simulink model "UAV_Simulation"  (R2021a)
settings: Solver=VariableStepAuto  StartTime=0.0  StopTime=100  RelTol=1e-3
libraries: pid_lib x4
settings Model: Creator=ewert  LastModifiedBy=varsh
settings SolverCC: AlgebraicLoopSolver=TrustRegion
settings DataIOCC: ReturnWorkspaceOutputs=off
settings DebuggingCC: SFMachineParentedDataDiag=warning  ArithmeticOperatorsInVariantConditions=warning
settings SFSimCC: SimUseLocalCustomCode=off  CustomCodeUndefinedFunction=UseInterfaceOnly
settings RTWCC: RTWUseLocalCustomCode=off
settings CodeAppCC: StateflowObjectComments=on

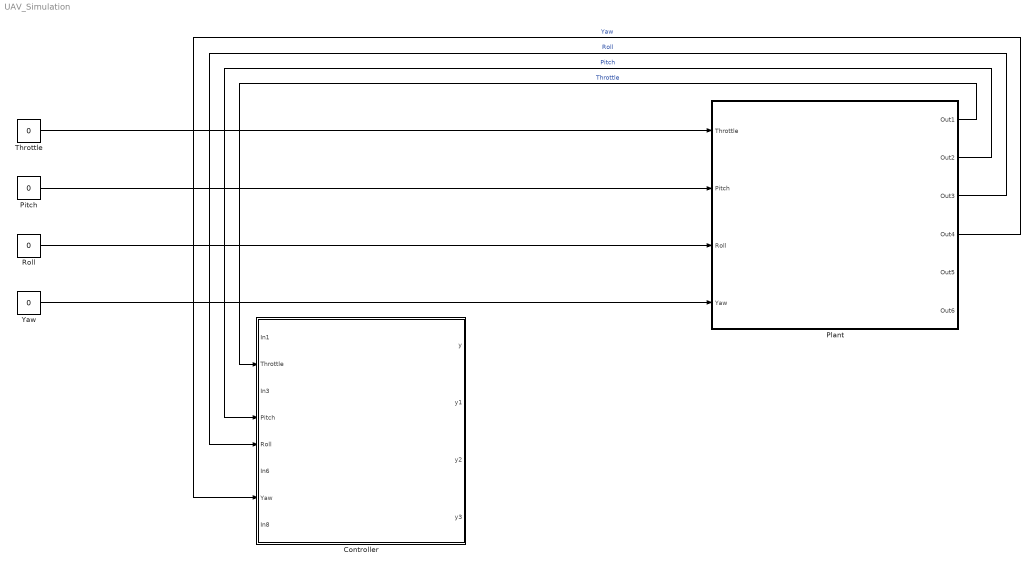
== system UAV_Simulation ==
  Controller : Subsystem
  Pitch : Constant  Value=0
  Plant : Subsystem
  Roll : Constant  Value=0
  Throttle : Constant  Value=0
  Yaw : Constant  Value=0
  wires:
  Plant/1(Out1) -> Controller/2(Throttle)  "Throttle"
  Plant/2(Out2) -> Controller/4(Pitch)  "Pitch"
  Plant/3(Out3) -> Controller/5(Roll)  "Roll"
  Plant/4(Out4) -> Controller/7(Yaw)  "Yaw"
  Roll/1 -> Plant/3(Roll)
  Yaw/1 -> Plant/4(Yaw)
  Throttle/1 -> Plant/1(Throttle)
  Pitch/1 -> Plant/2(Pitch)

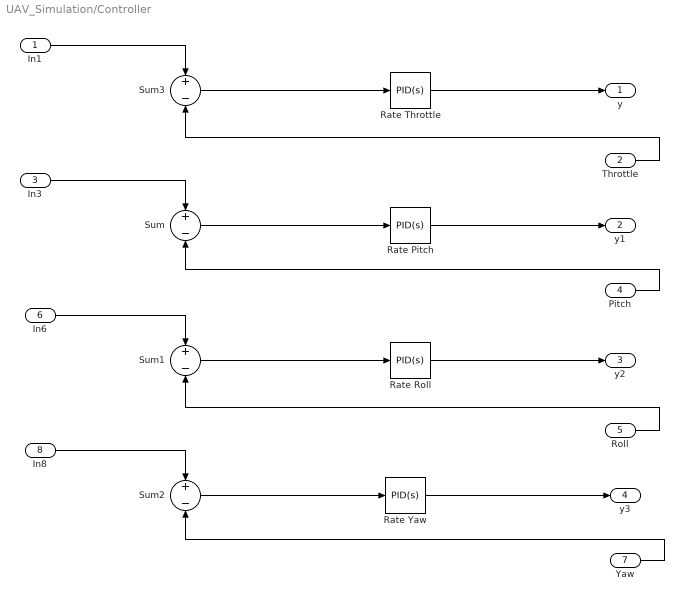
== system UAV_Simulation/Controller ==
  In1 : Inport
  Throttle : Inport  Port=2
  In3 : Inport  Port=3
  Pitch : Inport  Port=4
  Roll : Inport  Port=5
  In6 : Inport  Port=6
  Yaw : Inport  Port=7
  In8 : Inport  Port=8
  Rate Pitch : pid_lib/PID Controller  Controller=PID  Form=Parallel  TimeDomain=Continuous-time  UseExternalTs=off  SampleTime=-1  IntegratorMethod=Forward Euler  FilterMethod=Forward Euler  ControllerParametersSource=internal  P=5  I=1  D=0  UseFilter=on  N=100  TunerSelectOption=Transfer Function Based (PID Tuner App)  InitialConditionSource=internal  InitialConditionForIntegrator=0  InitialConditionForFilter=0  DifferentiatorICPrevScaledInput=0  ExternalReset=none  TrackingMode=off  Kt=1  LimitOutput=on  SatLimitsSource=internal  UpperSaturationLimit=100  LowerSaturationLimit=0  LinearizeAsGain=on  AntiWindupMode=clamping  Kb=1  POutMin=[]  POutMax=[]  IOutMin=[]  IOutMax=[]  DOutMin=[]  DOutMax=[]  NOutMin=[]  NOutMax=[]  SumOutMin=[]  SumOutMax=[]  SaturationOutMin=[]  SaturationOutMax=[]  PParamMin=[]  PParamMax=[]  IParamMin=[]  IParamMax=[]  DParamMin=[]  DParamMax=[]  NParamMin=[]  NParamMax=[]  KbParamMin=[]  KbParamMax=[]  KtParamMin=[]  KtParamMax=[]  KbOutMin=[]  KbOutMax=[]  KtOutMin=[]  KtOutMax=[]  IntegratorOutMin=[]  IntegratorOutMax=[]  FilterOutMin=[]  FilterOutMax=[]  SumI1OutMin=[]  SumI1OutMax=[]  SumI2OutMin=[]  SumI2OutMax=[]  SumI3OutMin=[]  SumI3OutMax=[]  SumI4OutMin=[]  SumI4OutMax=[]  SumDOutMin=[]  SumDOutMax=[]  DifferentiatorOutMin=[]  DifferentiatorOutMax=[]  FilterDiffOutCoefMin=[]  FilterDiffOutCoefMax=[]  ReciprocalOutMin=[]  ReciprocalOutMax=[]  SumDenOutMin=[]  SumDenOutMax=[]  SumNumOutMin=[]  SumNumOutMax=[]  DivideOutMin=[]  DivideOutMax=[]  UdiffTsProdOutMin=[]  UdiffTsProdOutMax=[]  NTsProdOutMin=[]  NTsProdOutMax=[]  UintegralTsProdOutMin=[]  UintegralTsProdOutMax=[]  UngainTsProdOutMin=[]  UngainTsProdOutMax=[]  IntegratorContinuousStateAttributes=''  IntegratorStateMustResolveToSignalObject=off  IntegratorRTWStateStorageClass=Auto  FilterContinuousStateAttributes=''  FilterStateMustResolveToSignalObject=off  FilterRTWStateStorageClass=Auto  ParallelPVariant=InternalParameters  IdealPVariant=Disabled  IVariant=InternalParameters  DVariant=InternalParameters  IntegratorVariant=Continuous  SatVariant=Enabled  AWVariant=ContClampingParallel  PCopyVariant=Disabled  TRVariant=Disabled  FdbkBlocksVariant=Forward  IdealPFdbkVariant=Disabled  SatFdbkVariant=Disabled  DerivativeFilterVariant=ContFilter  NVariant=InternalParameters  NCopyVariant=Disabled  FilterICVariant=InternalICsFilter  IntegratorICVariant=InternalICs  ExternalResetVariant=Disabled  TRSumVariant=Passthrough  SumFdbkVariant=Disabled  SumVariant=Sum_PID  TsampFilterVariant=InternalTs  TsampNgainVariant=Passthrough  TsampIntegralVariant=Passthrough  ExternalSaturationOutDataTypeStr=Inherit: Same as second input
  Rate Roll : pid_lib/PID Controller  Controller=PID  Form=Parallel  TimeDomain=Continuous-time  UseExternalTs=off  SampleTime=-1  IntegratorMethod=Forward Euler  FilterMethod=Forward Euler  ControllerParametersSource=internal  P=10  I=5  D=0  UseFilter=on  N=100  TunerSelectOption=Transfer Function Based (PID Tuner App)  InitialConditionSource=internal  InitialConditionForIntegrator=0  InitialConditionForFilter=0  DifferentiatorICPrevScaledInput=0  ExternalReset=none  TrackingMode=off  Kt=1  LimitOutput=on  SatLimitsSource=internal  UpperSaturationLimit=100  LowerSaturationLimit=0  LinearizeAsGain=on  AntiWindupMode=clamping  Kb=1  POutMin=[]  POutMax=[]  IOutMin=[]  IOutMax=[]  DOutMin=[]  DOutMax=[]  NOutMin=[]  NOutMax=[]  SumOutMin=[]  SumOutMax=[]  SaturationOutMin=[]  SaturationOutMax=[]  PParamMin=[]  PParamMax=[]  IParamMin=[]  IParamMax=[]  DParamMin=[]  DParamMax=[]  NParamMin=[]  NParamMax=[]  KbParamMin=[]  KbParamMax=[]  KtParamMin=[]  KtParamMax=[]  KbOutMin=[]  KbOutMax=[]  KtOutMin=[]  KtOutMax=[]  IntegratorOutMin=[]  IntegratorOutMax=[]  FilterOutMin=[]  FilterOutMax=[]  SumI1OutMin=[]  SumI1OutMax=[]  SumI2OutMin=[]  SumI2OutMax=[]  SumI3OutMin=[]  SumI3OutMax=[]  SumI4OutMin=[]  SumI4OutMax=[]  SumDOutMin=[]  SumDOutMax=[]  DifferentiatorOutMin=[]  DifferentiatorOutMax=[]  FilterDiffOutCoefMin=[]  FilterDiffOutCoefMax=[]  ReciprocalOutMin=[]  ReciprocalOutMax=[]  SumDenOutMin=[]  SumDenOutMax=[]  SumNumOutMin=[]  SumNumOutMax=[]  DivideOutMin=[]  DivideOutMax=[]  UdiffTsProdOutMin=[]  UdiffTsProdOutMax=[]  NTsProdOutMin=[]  NTsProdOutMax=[]  UintegralTsProdOutMin=[]  UintegralTsProdOutMax=[]  UngainTsProdOutMin=[]  UngainTsProdOutMax=[]  IntegratorContinuousStateAttributes=''  IntegratorStateMustResolveToSignalObject=off  IntegratorRTWStateStorageClass=Auto  FilterContinuousStateAttributes=''  FilterStateMustResolveToSignalObject=off  FilterRTWStateStorageClass=Auto  ParallelPVariant=InternalParameters  IdealPVariant=Disabled  IVariant=InternalParameters  DVariant=InternalParameters  IntegratorVariant=Continuous  SatVariant=Enabled  AWVariant=ContClampingParallel  PCopyVariant=Disabled  TRVariant=Disabled  FdbkBlocksVariant=Forward  IdealPFdbkVariant=Disabled  SatFdbkVariant=Disabled  DerivativeFilterVariant=ContFilter  NVariant=InternalParameters  NCopyVariant=Disabled  FilterICVariant=InternalICsFilter  IntegratorICVariant=InternalICs  ExternalResetVariant=Disabled  TRSumVariant=Passthrough  SumFdbkVariant=Disabled  SumVariant=Sum_PID  TsampFilterVariant=InternalTs  TsampNgainVariant=Passthrough  TsampIntegralVariant=Passthrough  ExternalSaturationOutDataTypeStr=Inherit: Same as second input
  Rate Throttle : pid_lib/PID Controller  Controller=PID  Form=Parallel  TimeDomain=Continuous-time  UseExternalTs=off  SampleTime=-1  IntegratorMethod=Forward Euler  FilterMethod=Forward Euler  ControllerParametersSource=internal  P=23.2003030381999  I=0.891787568643448  D=34.3816922508907  UseFilter=on  N=1142.8279760416  TunerSelectOption=Transfer Function Based (PID Tuner App)  InitialConditionSource=internal  InitialConditionForIntegrator=0  InitialConditionForFilter=0  DifferentiatorICPrevScaledInput=0  ExternalReset=none  TrackingMode=off  Kt=1  LimitOutput=on  SatLimitsSource=internal  UpperSaturationLimit=100  LowerSaturationLimit=0  LinearizeAsGain=on  AntiWindupMode=clamping  Kb=1  POutMin=[]  POutMax=[]  IOutMin=[]  IOutMax=[]  DOutMin=[]  DOutMax=[]  NOutMin=[]  NOutMax=[]  SumOutMin=[]  SumOutMax=[]  SaturationOutMin=[]  SaturationOutMax=[]  PParamMin=[]  PParamMax=[]  IParamMin=[]  IParamMax=[]  DParamMin=[]  DParamMax=[]  NParamMin=[]  NParamMax=[]  KbParamMin=[]  KbParamMax=[]  KtParamMin=[]  KtParamMax=[]  KbOutMin=[]  KbOutMax=[]  KtOutMin=[]  KtOutMax=[]  IntegratorOutMin=[]  IntegratorOutMax=[]  FilterOutMin=[]  FilterOutMax=[]  SumI1OutMin=[]  SumI1OutMax=[]  SumI2OutMin=[]  SumI2OutMax=[]  SumI3OutMin=[]  SumI3OutMax=[]  SumI4OutMin=[]  SumI4OutMax=[]  SumDOutMin=[]  SumDOutMax=[]  DifferentiatorOutMin=[]  DifferentiatorOutMax=[]  FilterDiffOutCoefMin=[]  FilterDiffOutCoefMax=[]  ReciprocalOutMin=[]  ReciprocalOutMax=[]  SumDenOutMin=[]  SumDenOutMax=[]  SumNumOutMin=[]  SumNumOutMax=[]  DivideOutMin=[]  DivideOutMax=[]  UdiffTsProdOutMin=[]  UdiffTsProdOutMax=[]  NTsProdOutMin=[]  NTsProdOutMax=[]  UintegralTsProdOutMin=[]  UintegralTsProdOutMax=[]  UngainTsProdOutMin=[]  UngainTsProdOutMax=[]  IntegratorContinuousStateAttributes=''  IntegratorStateMustResolveToSignalObject=off  IntegratorRTWStateStorageClass=Auto  FilterContinuousStateAttributes=''  FilterStateMustResolveToSignalObject=off  FilterRTWStateStorageClass=Auto  ParallelPVariant=InternalParameters  IdealPVariant=Disabled  IVariant=InternalParameters  DVariant=InternalParameters  IntegratorVariant=Continuous  SatVariant=Enabled  AWVariant=ContClampingParallel  PCopyVariant=Disabled  TRVariant=Disabled  FdbkBlocksVariant=Forward  IdealPFdbkVariant=Disabled  SatFdbkVariant=Disabled  DerivativeFilterVariant=ContFilter  NVariant=InternalParameters  NCopyVariant=Disabled  FilterICVariant=InternalICsFilter  IntegratorICVariant=InternalICs  ExternalResetVariant=Disabled  TRSumVariant=Passthrough  SumFdbkVariant=Disabled  SumVariant=Sum_PID  TsampFilterVariant=InternalTs  TsampNgainVariant=Passthrough  TsampIntegralVariant=Passthrough  ExternalSaturationOutDataTypeStr=Inherit: Same as second input
  Rate Yaw : pid_lib/PID Controller  Controller=PID  Form=Parallel  TimeDomain=Continuous-time  UseExternalTs=off  SampleTime=-1  IntegratorMethod=Forward Euler  FilterMethod=Forward Euler  ControllerParametersSource=internal  P=10  I=5  D=0  UseFilter=on  N=100  TunerSelectOption=Transfer Function Based (PID Tuner App)  InitialConditionSource=internal  InitialConditionForIntegrator=0  InitialConditionForFilter=0  DifferentiatorICPrevScaledInput=0  ExternalReset=none  TrackingMode=off  Kt=1  LimitOutput=on  SatLimitsSource=internal  UpperSaturationLimit=100  LowerSaturationLimit=0  LinearizeAsGain=on  AntiWindupMode=clamping  Kb=1  POutMin=[]  POutMax=[]  IOutMin=[]  IOutMax=[]  DOutMin=[]  DOutMax=[]  NOutMin=[]  NOutMax=[]  SumOutMin=[]  SumOutMax=[]  SaturationOutMin=[]  SaturationOutMax=[]  PParamMin=[]  PParamMax=[]  IParamMin=[]  IParamMax=[]  DParamMin=[]  DParamMax=[]  NParamMin=[]  NParamMax=[]  KbParamMin=[]  KbParamMax=[]  KtParamMin=[]  KtParamMax=[]  KbOutMin=[]  KbOutMax=[]  KtOutMin=[]  KtOutMax=[]  IntegratorOutMin=[]  IntegratorOutMax=[]  FilterOutMin=[]  FilterOutMax=[]  SumI1OutMin=[]  SumI1OutMax=[]  SumI2OutMin=[]  SumI2OutMax=[]  SumI3OutMin=[]  SumI3OutMax=[]  SumI4OutMin=[]  SumI4OutMax=[]  SumDOutMin=[]  SumDOutMax=[]  DifferentiatorOutMin=[]  DifferentiatorOutMax=[]  FilterDiffOutCoefMin=[]  FilterDiffOutCoefMax=[]  ReciprocalOutMin=[]  ReciprocalOutMax=[]  SumDenOutMin=[]  SumDenOutMax=[]  SumNumOutMin=[]  SumNumOutMax=[]  DivideOutMin=[]  DivideOutMax=[]  UdiffTsProdOutMin=[]  UdiffTsProdOutMax=[]  NTsProdOutMin=[]  NTsProdOutMax=[]  UintegralTsProdOutMin=[]  UintegralTsProdOutMax=[]  UngainTsProdOutMin=[]  UngainTsProdOutMax=[]  IntegratorContinuousStateAttributes=''  IntegratorStateMustResolveToSignalObject=off  IntegratorRTWStateStorageClass=Auto  FilterContinuousStateAttributes=''  FilterStateMustResolveToSignalObject=off  FilterRTWStateStorageClass=Auto  ParallelPVariant=InternalParameters  IdealPVariant=Disabled  IVariant=InternalParameters  DVariant=InternalParameters  IntegratorVariant=Continuous  SatVariant=Enabled  AWVariant=ContClampingParallel  PCopyVariant=Disabled  TRVariant=Disabled  FdbkBlocksVariant=Forward  IdealPFdbkVariant=Disabled  SatFdbkVariant=Disabled  DerivativeFilterVariant=ContFilter  NVariant=InternalParameters  NCopyVariant=Disabled  FilterICVariant=InternalICsFilter  IntegratorICVariant=InternalICs  ExternalResetVariant=Disabled  TRSumVariant=Passthrough  SumFdbkVariant=Disabled  SumVariant=Sum_PID  TsampFilterVariant=InternalTs  TsampNgainVariant=Passthrough  TsampIntegralVariant=Passthrough  ExternalSaturationOutDataTypeStr=Inherit: Same as second input
  Sum{,1..3} (4 alike) : Sum  Inputs=+-
  y : Outport
  y1 : Outport  Port=2
  y2 : Outport  Port=3
  y3 : Outport  Port=4
  wires:
  Rate Pitch/1 -> y1/1
  Sum/1 -> Rate Pitch/1
  Roll/1 -> Sum1/2
  In6/1 -> Sum1/1
  Sum1/1 -> Rate Roll/1
  Sum2/1 -> Rate Yaw/1
  In8/1 -> Sum2/1
  In3/1 -> Sum/1
  Sum3/1 -> Rate Throttle/1
  Rate Yaw/1 -> y3/1
  Rate Throttle/1 -> y/1
  Rate Roll/1 -> y2/1
  Yaw/1 -> Sum2/2
  Pitch/1 -> Sum/2
  In1/1 -> Sum3/1
  Throttle/1 -> Sum3/2

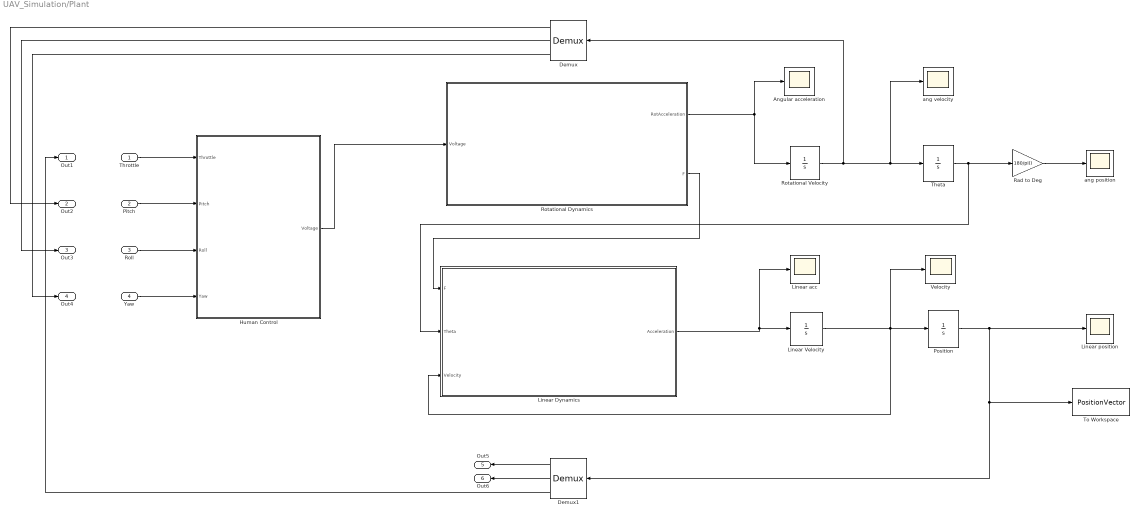
== system UAV_Simulation/Plant ==
  Throttle : Inport
  Pitch : Inport  Port=2
  Roll : Inport  Port=3
  Yaw : Inport  Port=4
  Angular acceleration : Scope
  Demux : Demux  Outputs=3
  Demux1 : Demux  Outputs=3
  Human Control : MATLAB Function  TreatAsAtomicUnit=on
  Linear Dynamics : Subsystem
  Linear Velocity : Integrator
  Linear acc : Scope
  Linear position : Scope
  Position : Integrator
  Rad to Deg : Gain  Gain=180/pi()
  Rotational Dynamics : Subsystem
  Rotational Velocity : Integrator
  Theta : Integrator
  To Workspace : ToWorkspace  VariableName=PositionVector  SampleTime=-1
      settings: Save2DSignal=2-D array (concatenate along first dimension)
  "Velocity " : Scope
  ang position : Scope
  ang velocity : Scope
  Out1 : Outport
  Out2 : Outport  Port=2
  Out3 : Outport  Port=3
  Out4 : Outport  Port=4
  Out5 : Outport  Port=5
  Out6 : Outport  Port=6
  wires:
  Linear Velocity/1 -> Linear Dynamics/3(Velocity), Position/1, "Velocity "/1
  Throttle/1 -> Human Control/1(Throttle)
  Demux1/1 -> Out5/1
  Demux/2 -> Out3/1
  Rotational Velocity/1 -> Theta/1, ang velocity/1, Demux/1
  Position/1 -> Demux1/1, To Workspace/1, Linear position/1
  Theta/1 -> Linear Dynamics/2(Theta), Rad to Deg/1
  Rad to Deg/1 -> ang position/1
  Pitch/1 -> Human Control/2(Pitch)
  Demux/1 -> Out2/1
  Demux1/3 -> Out1/1
  Roll/1 -> Human Control/3(Roll)
  Yaw/1 -> Human Control/4(Yaw)
  Demux/3 -> Out4/1
  Demux1/2 -> Out6/1
  Rotational Dynamics/1(RotAcceleration) -> Rotational Velocity/1, Angular acceleration/1
  Human Control/1(Voltage) -> Rotational Dynamics/1(Voltage)
  Linear Dynamics/1(Acceleration) -> Linear acc/1, Linear Velocity/1
  Rotational Dynamics/2(F) -> Linear Dynamics/1(F)

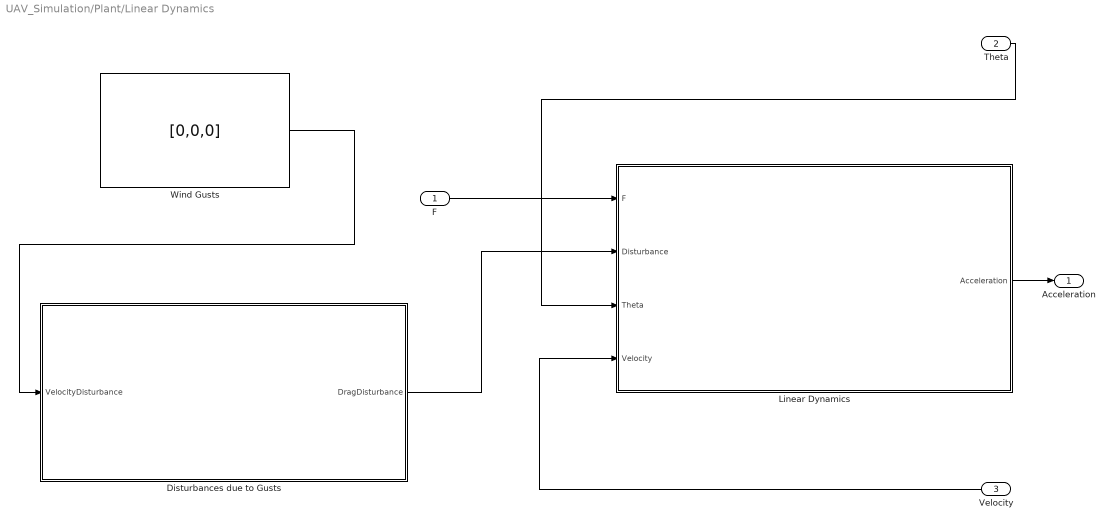
== system UAV_Simulation/Plant/Linear Dynamics ==
  F : Inport
  Theta : Inport  Port=2
  Velocity : Inport  Port=3
  Disturbances due to Gusts : MATLAB Function  TreatAsAtomicUnit=on
  Linear Dynamics : MATLAB Function  TreatAsAtomicUnit=on
  Wind Gusts : Constant  Value=[0,0,0]
  Acceleration : Outport
  wires:
  Disturbances due to Gusts/1(DragDisturbance) -> Linear Dynamics/2(Disturbance)
  Wind Gusts/1 -> Disturbances due to Gusts/1(VelocityDisturbance)
  Theta/1 -> Linear Dynamics/3(Theta)
  Velocity/1 -> Linear Dynamics/4(Velocity)
  F/1 -> Linear Dynamics/1(F)
  Linear Dynamics/1(Acceleration) -> Acceleration/1

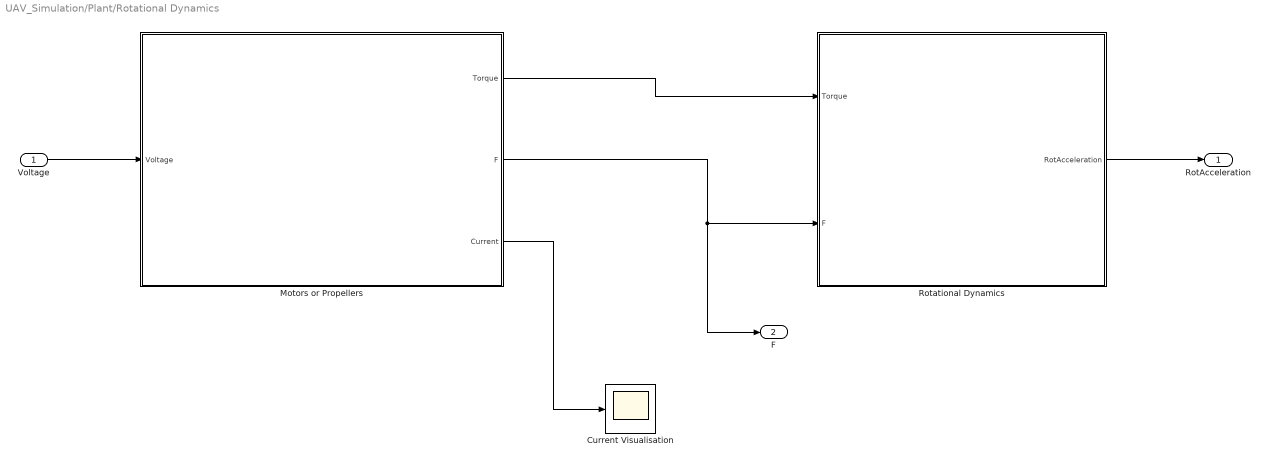
== system UAV_Simulation/Plant/Rotational Dynamics ==
  Voltage : Inport
  "Current Visualisation " : Scope
  Motors or Propellers : MATLAB Function  TreatAsAtomicUnit=on
  Rotational Dynamics : MATLAB Function  TreatAsAtomicUnit=on
  RotAcceleration : Outport
  F : Outport  Port=2
  wires:
  Motors or Propellers/2(F) -> F/1, Rotational Dynamics/2(F)
  Voltage/1 -> Motors or Propellers/1(Voltage)
  Motors or Propellers/3(Current) -> "Current Visualisation "/1
  Motors or Propellers/1(Torque) -> Rotational Dynamics/1(Torque)
  Rotational Dynamics/1(RotAcceleration) -> RotAcceleration/1

== matlab function UAV_Simulation/Plant/Rotational Dynamics/Rotational Dynamics ==
  data: Torque input; RotAcceleration output; F input
% from this we can work out rotational velocity and angle at which drone is at. 
% Calculate rotational acceleration in all 3 directions
function RotAcceleration = fcn(Torque, F)
Moment = [0 0 0]; % [x y z]
RotAcceleration = [0 0 0];
I = [0.003, 0.003, 0.007];

Moment(1) = (F(3) + F(4))*0.237/2 - (F(1) + F(2))*0.237/2;
Moment(2) = (F(3) + F(2))*0.237/2 - (F(1) + F(4))*0.237/2;

% clockwise torques and moments to be positive
Moment(3) = Torque(4) - Torque(1) + Torque(2) - Torque(3); 

for i = 1:3
    RotAcceleration(i) = Moment(i)/I(i);
end

== matlab function UAV_Simulation/Plant/Rotational Dynamics/Motors or Propellers ==
  data: Voltage input; Torque output; F output; Current output
function [Torque, F, Current] = fcn(Voltage)
RPM     = [0 0 0 0];
Torque  = [0 0 0 0];
Current = [0 0 0 0];
F       = [0 0 0 0];

for i = 1:4
    RPM(i) = -2.6931*Voltage(i)^3 + 1400*Voltage(i);
    
    % Coefficient of thrust
    Ct = 2*10^-15*RPM(i)^3 - 4*10^-11*RPM(i)^2 + 3*10^-7*RPM(i) + 0.1013;
    
    % Thrust produced by ith propeller (perpendicular to drone surface)
    F(i) = Ct*1.225*(RPM(i)/60)^2*0.2^4;
    
    % Torque produced by ith propeller
    Torque(i) = 4*10^-14*RPM(i)^3 + 8*10^-12*RPM(i)^2 + 3*10^-6*RPM(i);
    
    Current(i) = 1400 * Torque(i);
end

== matlab function UAV_Simulation/Plant/Linear Dynamics/Linear Dynamics ==
  data: F input; Acceleration output; Disturbance input; Theta input; Velocity input
% Velocity: linear, Acceleration: linear
function Acceleration  = fcn(F, Disturbance, Theta, Velocity)

% m is mass of the drone
m = 0.743;

% g is acceleration due to gravity
g = 9.81;

% A is area of the drone in x, y, z axis
A = [0.0197 0.0197 0.0512];

rho = 1.225;
Cd = 1;

Acceleration = [0 0 0];
Force = [0 0 0];
Fprop = [0;0;0];

% Calculate thrust created by propeller in x, y, z direction
Fprop(1,1) = sin(Theta(2))*cos(Theta(1))*(F(1) + F(2) + F(3) + F(4));
Fprop(2,1) = sin(Theta(1))*cos(Theta(2))*(F(1) + F(2) + F(3) + F(4));
Fprop(3,1) = (F(1) + F(2) + F(3) + F(4))*cos(Theta(1))*cos(Theta(2));

ThetaXY = -atan2(Fprop(1), Fprop(2));

% magnitude of projection of thrust vector on XY plane:
XY2D = sqrt(Fprop(1)^2 + Fprop(2)^2);

% drone is pointing upwards
if Fprop(3) >= 0
    Fprop(1) = XY2D*sin(Theta(3) + ThetaXY);
    Fprop(2) = XY2D*cos(Theta(3) + ThetaXY);
else
    Fprop(1) = XY2D*sin(-Theta(3) + ThetaXY);
    Fprop(2) = XY2D*cos(-Theta(3) + ThetaXY);
end
    
% if drag acts in opposite direction of motion
if Velocity(1) < 0
    Force(1) = Fprop(1) - Disturbance(1) + 0.5*rho*Velocity(1)^2*A(1)*Cd;
else 
    Force(1) = Fprop(1) - Disturbance(1) - 0.5*rho*Velocity(1)^2*A(1)*Cd;
end

if Velocity(2)<0
    Force(2) = Fprop(2) - Disturbance(2) + 0.5*rho*Velocity(2)^2*A(2)*Cd;
else 
    Force(2) = Fprop(2) - Disturbance(2) - 0.5*rho*Velocity(2)^2*A(2)*Cd;
end

if Velocity(3) < 0
    Force(3) = Fprop(3) + 0.5*rho*Velocity(3)^2*A(3)*Cd - m*g - Disturbance(3);
else 
    Force(3) = Fprop(3) - 0.5*rho*Velocity(3)^2*A(3)*Cd - m*g - Disturbance(3);
end

for i = 1:3
    Acceleration(i) = Force(i)/m;
end

== matlab function UAV_Simulation/Plant/Linear Dynamics/Disturbances due to Gusts ==
  data: VelocityDisturbance input; DragDisturbance output
function DragDisturbance = fcn(VelocityDisturbance)
A = [0.0197 0.0197 0.0197*2*1.3];
DragDisturbance = [0 0 0];
rho = 1.225;
Cd = 1;

% wind gusts are in meter per second 
% force applied on drone by gust
for i = 1:3
    % check direction of gust
    if VelocityDisturbance(i) < 0
        DragDisturbance(i) = 0.5*rho*VelocityDisturbance(i)^2*A(i)*Cd;
    else
        DragDisturbance(i) = -0.5*rho*VelocityDisturbance(i)^2*A(i)*Cd;
    end
end

== matlab function UAV_Simulation/Plant/Human Control ==
  data: Throttle input; Voltage output; Pitch input; Roll input; Yaw input
% pitch, roll and yaw should be >= 0
% if everything is going to be throttle then there will not be pitch, roll and yaw
function Voltage = fcn(Throttle, Pitch, Roll, Yaw)
Correct = 0;
if (Pitch/2 + Roll/2 + Yaw/2 + Throttle) > 100
    Correct = (Pitch/2 + Roll/2 + Yaw/2 + Throttle - 100);
end

% drone will not be able to compensate for it's own weight if this condition is false
% propellers should not have 0 power
if (Pitch/2 + Roll/2 + Yaw/2) > (Throttle)
    if Correct < ((Pitch/2 + Roll/2 + Yaw/2) - (Throttle))
       Correct = ((Pitch/2 + Roll/2 + Yaw/2) - (Throttle));
    end
end

% our total signal should stays within 100 percent at the end
% that makes sense ask not more than 100 percent from motors
% factors on correct to be relevant to the comparisons above which look at the actual application
% subtracting the excess signal evenly
if Correct ~= 0
    Pitch = Pitch - Correct/3*2;
    Roll = Roll - Correct/3*2;
    Yaw = Yaw - Correct/3*2;
end

% we will not ask more than 100 percent from the motors and not less than 0 percent from the motors
% to make voltage, since these are in terms of percentage divide them by 100
% to get +ve pitch, decrease motor 1 and 2 and increase 3 and 4

% system doesn't go below 0 percent and above 100 percent on any of the propellers
Voltage=[(Throttle - Pitch/2 - Roll/2 - Yaw/2)*11.4/100 
    (Throttle - Pitch/2 + Roll/2 + Yaw/2)*11.4/100
    (Throttle + Pitch/2 + Roll/2 - Yaw/2)*11.4/100
    (Throttle + Pitch/2 - Roll/2 + Yaw/2)*11.4/100
];
